simulink model "message2"  (R2023a)
settings: Solver=VariableStepDiscrete  StartTime=0.0  StopTime=0.5  RelTol=1e-3
PreLoadFcn:
  | load sbit
InitFcn:
  | frameLength = 200;
  | numDelayCalcs = 3;
libraries: commseqgen3 x2, dspstat3 x2, commutil2 x2, commdigbbndpm3 x2, simulink x1, dspbuff3 x1, dspmathops x1, dspsrcs4 x1
CloseFcn:
  | clear frameLength numDelayCalcs
settings Model: Creator=mmclerno  LastModifiedBy=ascolwell
settings SolverCC: AlgebraicLoopSolver=TrustRegion
settings DataIOCC: LimitDataPoints=on  SaveFormat=Array  SignalLoggingSaveFormat=ModelDataLogs  SaveOutput=off  SaveTime=off  ReturnWorkspaceOutputs=off
settings OptimizationCC: BooleanDataType=off  DefaultParameterBehavior=Inlined  ExpressionDepthLimit=2147483647  LocalBlockOutputs=off  LifeSpan=inf
settings DebuggingCC: AlgebraicLoopMsg=error  UnderspecifiedInitializationDetection=Classic  MergeDetectMultiDrivingBlocksExec=none  SolverPrmCheckMsg=warning  SingleTaskRateTransMsg=error  FcnCallInpInsideContextMsg=warning  UnconnectedInputMsg=warning  UnconnectedOutputMsg=warning  UnconnectedLineMsg=warning  StateNameClashWarn=warning  SFUnexpectedBacktrackingDiag=warning  SFNoUnconditionalDefaultTransitionDiag=warning  SFExecutionAtInitializationDiag=none  ArithmeticOperatorsInVariantConditions=warning
settings HardwareCC: ProdBitPerPointer=32  ProdBitPerSizeT=32  ProdBitPerPtrDiffT=32  ProdLargestAtomicFloat=None  ProdIntDivRoundTo=Undefined  ProdEndianess=Unspecified  ProdWordSize=32  ProdHWDeviceType=32-bit Generic
settings ModelReferenceCC: PropagateSignalLabelsOutOfModel=off
settings SFSimCC: SimUseLocalCustomCode=off  CustomCodeUndefinedFunction=UseInterfaceOnly
settings RTWCC: RTWUseLocalCustomCode=off
settings CodeAppCC: StateflowObjectComments=on
settings GRTTargetCC: TargetLangStandard=C89/C90 (ANSI)  CombineOutputUpdateFcns=off  GRTInterface=on
settings ConfigComp: CovMetricSettings=dw  CovSaveCumulativeToWorkspaceVar=on  CovSaveSingleToWorkspaceVar=on  CovExternalEMLEnable=off  CovSFcnEnable=off

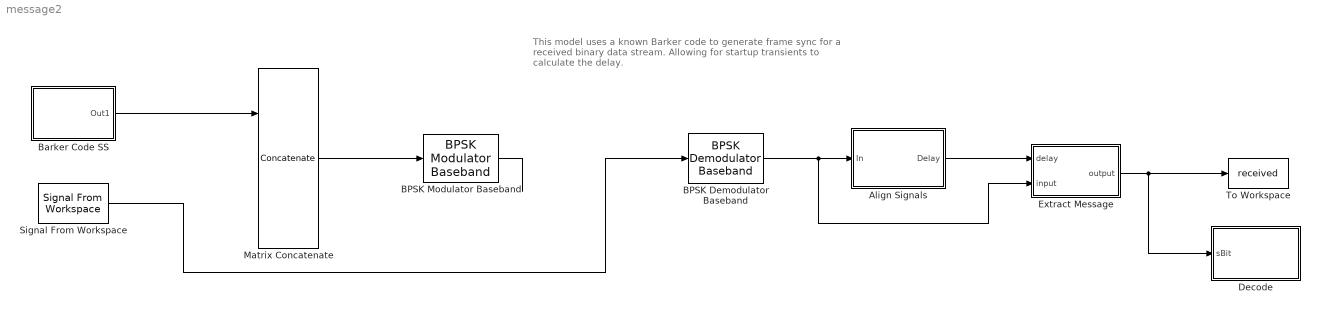
== system message2 ==
  note: This model uses a known Barker code to generate frame sync
      | for a received binary data stream.  Allowing for startup transients
      | to calculate the delay.
  Align Signals : Subsystem
  BPSK Demodulator Baseband : commdigbbndpm3/BPSK Demodulator Baseband  DecType=Hard decision  VarSource=Dialog  Variance=1  Ph=0  outDtype=Inherit via internal rule  derotateFactorWordLen=16  derotateFactorDataTypeStr=Inherit: Same word length as input  derotateFactorLastDataTypeStr=Inherit: Same word length as input
  BPSK Modulator Baseband : commdigbbndpm3/BPSK Modulator Baseband  Ph=0  outDtype=double  outWordLen=16  outUDDataType=sfix(16)  outFracLenMode=Best precision  outFracLen=15  outDataTypeStr=double  outLastDataTypeStr=double
  Barker Code SS : Subsystem
      mask Display: disp('Unipolar\nBarker Code')
  "Decode " : MATLAB Function  TreatAsAtomicUnit=on
  "Extract Message " : MATLAB Function  TreatAsAtomicUnit=on
  Matrix Concatenate : Concatenate  Mode=Multidimensional array
  Signal From Workspace : dspsrcs4/Signal From Workspace  X=info  Ts=1/(122 + 7)  nsamps=(112+7)  OutputAfterFinalValue=Cyclic repetition  ignoreOrWarnInputAndFrameLengths=off  OutputFrames=on
  To Workspace : ToWorkspace  VariableName=received  SampleTime=-1
  wires:
  Barker Code SS/1(Out1) -> Matrix Concatenate/1
  Matrix Concatenate/1 -> BPSK Modulator Baseband/1
  BPSK Modulator Baseband/1 -> ?
  Signal From Workspace/1 -> BPSK Demodulator Baseband/1
  BPSK Demodulator Baseband/1 -> Align Signals/1(In), "Extract Message "/2(input)
  Align Signals/1(Delay) -> "Extract Message "/1(delay)
  "Extract Message "/1(output) -> To Workspace/1, "Decode "/1(sBit)

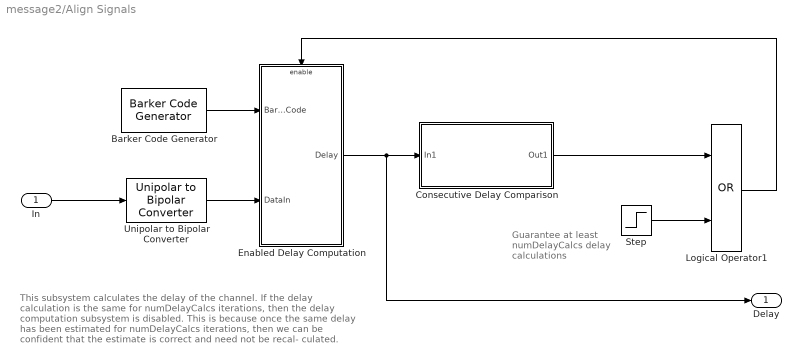
== system message2/Align Signals ==
  note: This subsystem calculates the delay of the channel.  If the delay
      | calculation is the same for numDelayCalcs iterations, then the delay
      | computation subsystem is disabled.  This is because once the same
      | delay has been estimated for numDelayCalcs iterations, then we
      | can be confident that the estimate is correct and need not be recal-
      | culated.
  note: Guarantee at least
      | numDelayCalcs delay
      | calculations
  In : Inport
  Barker Code Generator : commseqgen3/Barker Code Generator  Length=7  LengthSimulink=7  SampleTime=1/7  SamplesPerFrame=7  OutputDataType=double  SimulateUsing=Code generation
  Consecutive Delay Comparison : Subsystem
      mask Display: disp('Compute Whether\nnumDelayCalcsDelay\nComputations Are\nIdentical')
  Enabled Delay Computation : Subsystem  TreatAsAtomicUnit=on
  Logical Operator1 : Logic  Operator=OR  AllPortsSameDT=off  OutDataTypeStr=boolean
  Step : Step  Time=numDelayCalcs-1  Before=1  After=0  SampleTime=1
  Unipolar to Bipolar Converter : commutil2/Unipolar to Bipolar Converter  M=2  polarity=Positive  dataType=Inherit via internal rule
  Delay : Outport
  wires:
  Barker Code Generator/1 -> Enabled Delay Computation/1(Barker Code)
  Enabled Delay Computation/1(Delay) -> Consecutive Delay Comparison/1(In1), Delay/1
  In/1 -> Unipolar to Bipolar Converter/1
  Unipolar to Bipolar Converter/1 -> Enabled Delay Computation/2(DataIn)
  Consecutive Delay Comparison/1(Out1) -> Logical Operator1/1
  Step/1 -> Logical Operator1/2
  Logical Operator1/1 -> Enabled Delay Computation/Enable

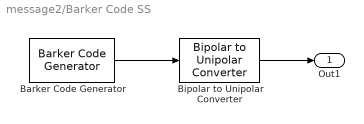
== system message2/Barker Code SS ==
  Barker Code Generator : commseqgen3/Barker Code Generator  Length=7  LengthSimulink=13  SampleTime=1/13  SamplesPerFrame=13  OutputDataType=double  SimulateUsing=Code generation
  Bipolar to Unipolar Converter : commutil2/Bipolar to Unipolar Converter  M=2  polarity=Positive  dataType=Inherit via internal rule
  Out1 : Outport
  wires:
  Barker Code Generator/1 -> Bipolar to Unipolar Converter/1
  Bipolar to Unipolar Converter/1 -> Out1/1

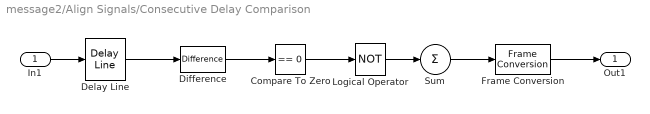
== system message2/Align Signals/Consecutive Delay Comparison ==
  In1 : Inport
  Compare To Zero : simulink/Logic and Bit Operations/Compare To Zero  relop===  OutDataTypeStr=uint8
  Delay Line : dspbuff3/Delay Line  siz=numDelayCalcs  ic=0  directfeed=off  enable_output=off  hold_output=off  OutputFrames=on
  Difference : dspmathops/Difference  Run=No  dim=Columns  Dimension=1  roundingMode=Floor  overflowMode=off  outputDataTypeStr=Inherit: Same as accumulator  outputMin=[]  outputMax=[]  outputLastDataTypeStr=Inherit: Same as accumulator
  Frame Conversion : FrameConversion  OutFrame=Sample-based
  Logical Operator : Logic  Operator=NOT  AllPortsSameDT=off  OutDataTypeStr=boolean
  Sum : Sum  Inputs=+
  Out1 : Outport
  wires:
  Delay Line/1 -> Difference/1
  Difference/1 -> Compare To Zero/1
  Compare To Zero/1 -> Logical Operator/1
  Frame Conversion/1 -> Out1/1
  Sum/1 -> Frame Conversion/1
  In1/1 -> Delay Line/1
  Logical Operator/1 -> Sum/1

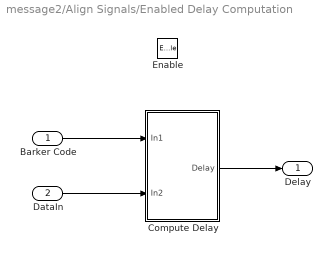
== system message2/Align Signals/Enabled Delay Computation ==
  Barker Code : Inport
  DataIn : Inport  Port=2
  Enable : EnablePort
  Compute Delay : Subsystem
      mask Display: disp('Compute\nDelay')
  Delay : Outport
  wires:
  Barker Code/1 -> Compute Delay/1(In1)
  DataIn/1 -> Compute Delay/2(In2)
  Compute Delay/1(Delay) -> Delay/1

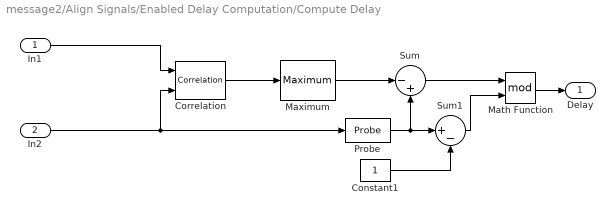
== system message2/Align Signals/Enabled Delay Computation/Compute Delay ==
  In1 : Inport
  In2 : Inport  Port=2
  Constant1 : Constant  VectorParams1D=off  OutDataTypeStr=Inherit: Inherit via back propagation  FramePeriod=2
  Correlation : dspstat3/Correlation  domain=Time  roundingMode=Floor  overflowMode=off  accumDataTypeStr=Inherit: Same as product output  accumLastDataTypeStr=Inherit: Same as product output  outputDataTypeStr=Inherit: Same as accumulator  outputMin=[]  outputMax=[]  outputLastDataTypeStr=Inherit: Same as accumulator
  Math Function : Math  Operator=mod  SignedPower=on
  Maximum : dspstat3/Maximum  operation=maximum  fcn=Index  indexBase=One  operateOver=Each column  Dimension=1  InputProcessing=Columns as channels (frame based)  reset=None  roiEnable=off  roiType=Rectangles  roiPortion=Entire ROI  roiOutput=Individual statistics for each ROI  roiFlag=off  roundingMode=Floor  overflowMode=off  accumDataTypeStr=Inherit: Same as product output  accumLastDataTypeStr=Inherit: Same as product output
  Probe : Probe  ProbeSampleTime=off  ProbeComplexSignal=off
  Sum : Sum  Inputs=|-+  InputSameDT=on  SaturateOnIntegerOverflow=on  OutDataTypeStr=Inherit: Same as first input
  Sum1 : Sum  Inputs=|+-  InputSameDT=on  SaturateOnIntegerOverflow=on  OutDataTypeStr=Inherit: Same as first input
  Delay : Outport
  wires:
  Constant1/1 -> Sum1/2
  Sum1/1 -> Math Function/2
  Math Function/1 -> Delay/1
  Sum/1 -> Math Function/1
  Probe/1 -> Sum1/1, Sum/2
  Maximum/1 -> Sum/1
  In2/1 -> Probe/1, Correlation/2
  In1/1 -> Correlation/1
  Correlation/1 -> Maximum/1

== matlab function message2/Extract Message  ==
  data: delay input; input input; output output
function output = fcn(delay,input)
%#codegen

output = input(delay+7+1:delay+7+112);

== matlab function message2/Decode  ==
  data: sBit input
function  fcn(sBit)

%Convert bit stream back to integers
sBit = reshape(sBit, 7, 16);
sBit = sBit';
sIntEst = bi2de(sBit, 'left-msb');

%Convert integers back to characters
sEst = (char(sIntEst))'
end
